simulink library "aerolibwind"  (Simulink 5.0)
libraries: simulink x2, aerolibutil x1
settings Model: ForwardingTableString=||__slOldName__||aerolibwind/Dryden Wind Turbulence Model||__slNewName__||aerolibprivatev1p5/Dryden Wind Turbulence Model||__slOldName__||aerolibwind/Discrete Wind Gust Model||__slNewName__||aerolibprivatev1p5/Discrete Wind Gust Model||__slOldName__||aerolibwind/Wind Shear Model||__slNewName__||aerolibprivatev1p5/Wind Shear Model  Creator=sgage  LastModifiedBy=sgage  ExtModeAutoUpdateStatusClock=off  TargetHWChar=2  TargetHWWordLengths=8,16,32,32

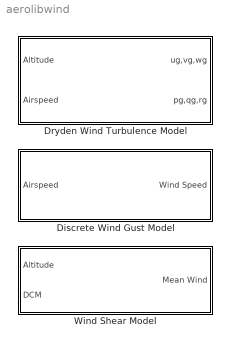
== system aerolibwind ==
  Discrete Wind Gust Model : Subsystem  mask(Discrete Wind Gust Model){v_units=meters/second, Gx=on, Gy=on, Gz=on, t_0=5, d_m=[120 120 80], v_m=[3.5 3.5 3.0]}
      mask prompts: v_units "Units of velocity:"; Gx "Check for gust in u-axis"; Gy "Check for gust in v-axis"; Gz "Check for gust in w-axis"; t_0 "Gust start time (seconds):"; d_m "Gust length [dx dy dz] (meters):"; v_m "Gust amplitude [ug vg wg] (meters/second):"
      mask help: Generate a discrete wind gust. The gust profile takes the '1-cosine' form.
      mask init:
      | m2ft= 3.28084;
      | mps2knot=1.94384;
      | if strcmp(v_units, 'meters/second')
      |   gust_units=1;
      |   mask_text1='m';
      |   mask_text2='m/s';
      | elseif strcmp(v_units, 'feet/second')
      |   gust_units=1;
      |   mask_text1='ft';
      |   mask_text2='ft/s';
      | else
      |   gust_units=m2ft/mps2knot;
      |   mask_text1='ft';
      |   mask_text2='knots';
      | end
      mask Help: web(asbhelp);
      mask StyleString: popup(meters/second|feet/second|knots),checkbox,checkbox,checkbox,edit,edit,edit
      mask CallbackString: aeroicon('aeroblkwindgust')||||||
      mask Display:
      | port_label('output', 1, ['Wind velocity (', mask_text2, ')'])
      | port_label('input', 1, ['Airspeed (', mask_text2, ')'])
  Dryden Wind Turbulence Model : Subsystem  mask(Dryden Wind Turbulence Model){v_units=meters/second, W20=15, TurbProb=10^-2 - Light, L_high=533, Wingspan=10, ts=0.1, Seed=[23341 23342 23343 23344], T_on=on}
      mask prompts: v_units "Units of velocity:"; W20 "Wind speed at 6 m defines the low-altitude intensity (meters/second):"; TurbProb "Probability of exceedance of high-altitude intensity"; L_high "Scale length at medium/high altitudes (meters):"; Wingspan "Wingspan (meters):"; ts "Band-limited noise sample time (seconds):"; Seed "Noise seeds [ug vg wg pg]:"; T_on "Turbulence on"
      mask help: Generate atmospheric turbulence. White noise is passed through a filter to give the turbulence the Dryden velocity spectra.
      mask init:
      | h_vec = [.5 1.75 3.75 7.5 15 25 35 45 55 65 75 80]*1000;% feet
      | sigma_vec(1,:) = [3.2 2.2 1.5 zeros(1,9)]; % ft/sec
      | sigma_vec(2,:) = [4.2 3.6 3.3 1.6 zeros(1,8)];
      | sigma_vec(3,:) = [6.6 6.9 7.4 6.7 4.6 2.7 0.4 zeros(1,5)];
      | sigma_vec(4,:) = [8.6 9.6 10.6 10.1 8.0 6.6 5.0 4.2 2.7 zeros(1,3)];
      | sigma_vec(5,:) = [11.8 13.0 16.0 15.1 11.6 9.7 8.1 8.2 7.9 4.9 3.2 2.1];
      | sigma_vec(6,:) = [15.6 17.6 23.0 23.6 22.1 20.0 16.0 15.1 12.1 7.9 6.2 5.1];
      | sigma_vec(7,:) = [18.7 21.5 28.4 30.2 30.7 31.0 25.2 23.1 17.5 10.7 8.4 7.2];
      | m2ft= 3.28084;
      | mps2knot=1.94384;
      | max_height_low = 1000;
      | min_height_high = 2000;
      | if strcmp(v_units, 'meters/second')
      |     gust_units=1;
      |     alt_units = m2ft;
      |     mask_text1='m';
      |     mask_text2='m/s';
      |     h_vec = h_vec/m2ft;
      |     sigma_vec = sigma_vec/m2ft;
      |     max_height_low = 1000/m2ft;
      |     min_height_high = 2000/m2ft;
      | elseif strcmp(v_units, 'feet/second')
      |     gust_units=1;
      |     alt_units =1;
      |     mask_text1='ft';
      |     mask_text2='ft/s';
      | else
      |     gust_units=m2ft/mps2knot;
      |     alt_units=1;
      |     mask_text1='ft';
      |     mask_text2='knots';
      | end
      mask Help: web(asbhelp);
      mask StyleString: popup(meters/second|feet/second|knots),edit,popup(2x10^-1|10^-1|10^-2 - Light |10^-3 - Moderate|10^-4|10^-5 - Severe|10^-6),edit,edit,edit,edit,checkbox
      mask CallbackString: aeroicon('aeroblkwindturb')|||||||
      mask Display:
      | port_label('output', 1, [' Wind velocity  (', mask_text2, ')'])
      | port_label('output', 2, 'Angular rates (rad/sec)')
      | port_label('input', 1, ['Altitude (', mask_text1, ')'])
      | port_label('input', 2, ['Airspeed (', mask_text2, ')'])
  Wind Shear Model : Subsystem  mask(Wind Shear Model){v_units=meters/second, phase=Category C - Terminal Flight Phase, W_20=15, Wdeg=0}
      mask prompts: v_units "Units of velocity:"; phase "Flight phase:"; W_20 "Wind speed at 6 meters altitude (meters/second):"; Wdeg "Wind direction at 6 meters altitude (degrees clockwise from north):"
      mask help: Calculate the wind shear from conditions measured at a height of 6 meters (20 feet) above the ground.
      mask init:
      | m2ft= 3.28084;
      | if strcmp(v_units, 'meters/second')
      |   if phase == 1;z0 = 0.15/m2ft;else;z0=2.0/m2ft;end;
      |   min_height = 3/m2ft;
      |   ref_height = 6;
      |   mask_text1='m';
      |   mask_text2='m/s';
      | elseif strcmp(v_units, 'feet/second')
      |   if phase == 1;z0 = 0.15;else;z0=2.0;end;
      |   min_height = 3;
      |   ref_height = 20;
      |   mask_text1='ft';
      |   mask_text2='ft/s';
      | else
      |   if phase == 1;z0 = 0.15;else;z0=2.0;end;
      |   min_height = 3;
      |   ref_height = 20;
      |   mask_text1='ft';
      |   mask_text2='knots';
      | end
      mask Help: web(asbhelp);
      mask StyleString: popup(meters/second|feet/second|knots),popup(Category C - Terminal Flight Phase|Other),edit,edit
      mask CallbackString: aeroicon('aeroblkwindshear')|||
      mask Display:
      | port_label('output', 1, ['Wind velocity (', mask_text2, ')'])
      | port_label('input', 1, ['Altitude (', mask_text1, ')'])
      | port_label('input', 2, 'DCM')

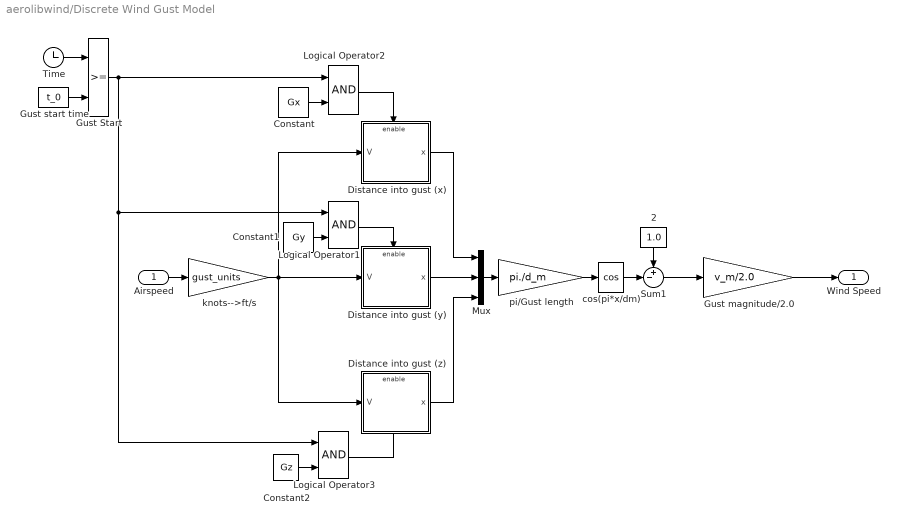
== system aerolibwind/Discrete Wind Gust Model ==
  Airspeed : Inport
  2 : Constant  Orientation=down  Value=1.0
  Constant : Constant  Value=Gx
  Constant1 : Constant  Value=Gy
  Constant2 : Constant  Value=Gz
  Distance into gust (x) : Subsystem  TreatAsAtomicUnit=on  mask{d_m=d_m(1)}
      mask prompts: d_m "Gust length d:"
  Distance into gust (y) : Subsystem  TreatAsAtomicUnit=on  mask{d_m=d_m(2)}
      mask prompts: d_m "Gust length d:"
  Distance into gust (z) : Subsystem  TreatAsAtomicUnit=on  mask{d_m=d_m(3)}
      mask prompts: d_m "Gust length d:"
  Gust Start : RelationalOperator  ShowAdditionalParam=on  LogicOutDataTypeMode=Specify via dialog  LogicDataType=float('double')  InputSameDT=on
  Gust magnitude/2.0 : Gain  Gain=v_m/2.0  SaturateOnIntegerOverflow=on
  Gust start time : Constant  Value=t_0
  Logical Operator1 : Logic  ShowAdditionalParam=on  AllPortsSameDT=off
  Logical Operator2 : Logic  ShowAdditionalParam=on  AllPortsSameDT=off
  Logical Operator3 : Logic  ShowAdditionalParam=on  AllPortsSameDT=off
  Mux : Mux  Inputs=3
  Sum1 : Sum  Inputs=+-|  SaturateOnIntegerOverflow=on  InputSameDT=on
  Time : Clock
      settings: Decimation=10
  cos(pi*x/dm) : Trigonometry  Operator=cos
  knots-->ft/s : Gain  Gain=gust_units  SaturateOnIntegerOverflow=on
  pi/Gust length : Gain  Gain=pi./d_m  SaturateOnIntegerOverflow=on
  Wind Speed : Outport
  wires:
  knots-->ft/s/1 -> Distance into gust (z)/1(V), Distance into gust (x)/1(V), Distance into gust (y)/1(V)
  Distance into gust (x)/1(x) -> Mux/1
  Constant/1 -> Logical Operator2/2
  Gust Start/1 -> Logical Operator2/1, Logical Operator3/1, Logical Operator1/1
  Airspeed/1 -> knots-->ft/s/1
  Logical Operator2/1 -> Distance into gust (x)/Enable
  Constant1/1 -> Logical Operator1/2
  Logical Operator1/1 -> Distance into gust (y)/Enable
  Constant2/1 -> Logical Operator3/2
  Logical Operator3/1 -> Distance into gust (z)/Enable
  Mux/1 -> pi/Gust length/1
  Distance into gust (z)/1(x) -> Mux/3
  Distance into gust (y)/1(x) -> Mux/2
  Gust start time/1 -> Gust Start/2
  Time/1 -> Gust Start/1
  Gust magnitude/2.0/1 -> Wind Speed/1
  cos(pi*x/dm)/1 -> Sum1/2
  Sum1/1 -> Gust magnitude/2.0/1
  2/1 -> Sum1/1
  pi/Gust length/1 -> cos(pi*x/dm)/1

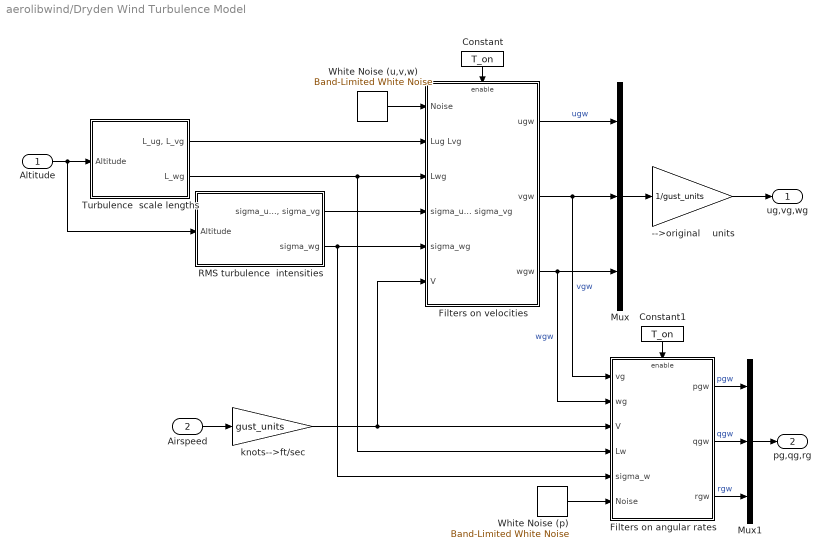
== system aerolibwind/Dryden Wind Turbulence Model ==
  Altitude : Inport
  Airspeed : Inport  Port=2
  -->original    units : Gain  Gain=1/gust_units  SaturateOnIntegerOverflow=on
  Constant : Constant  Orientation=down  Value=T_on
  Constant1 : Constant  Orientation=down  Value=T_on
  Filters on angular rates : Subsystem  TreatAsAtomicUnit=on
  Filters on velocities : Subsystem  TreatAsAtomicUnit=on
  Mux : Mux  Inputs=3
  Mux1 : Mux  Inputs=3
  RMS turbulence  intensities : Subsystem
  Turbulence  scale lengths : Subsystem
  White Noise (p) : simulink/Sources/Band-Limited White Noise  Cov=1  Ts=ts  seed=Seed(4)
  White Noise (u,v,w) : simulink/Sources/Band-Limited White Noise  Cov=[1 1 1]  Ts=ts  seed=Seed(1:3)
  knots-->ft/sec : Gain  Gain=gust_units  SaturateOnIntegerOverflow=on
  ug,vg,wg : Outport
  pg,qg,rg : Outport  Port=2
  wires:
  Constant1/1 -> Filters on angular rates/Enable
  Constant/1 -> Filters on velocities/Enable
  Filters on velocities/3(wgw) -> Filters on angular rates/2(wg), Mux/3  "wgw"
  Filters on velocities/2(vgw) -> Filters on angular rates/1(vg), Mux/2  "vgw"
  RMS turbulence  intensities/1("sigma_ug, sigma_vg ") -> Filters on velocities/4(sigma_ug sigma_vg)
  Filters on velocities/1(ugw) -> Mux/1  "ugw"
  Filters on angular rates/3(rgw) -> Mux1/3  "rgw"
  Filters on angular rates/2(qgw) -> Mux1/2  "qgw"
  Filters on angular rates/1(pgw) -> Mux1/1  "pgw"
  Mux1/1 -> pg,qg,rg/1
  Mux/1 -> -->original    units/1
  RMS turbulence  intensities/2(sigma_wg) -> Filters on velocities/5(sigma_wg), Filters on angular rates/5(sigma_w)
  Turbulence  scale lengths/2(L_wg) -> Filters on angular rates/4(Lw), Filters on velocities/3(Lwg)
  Turbulence  scale lengths/1("L_ug, L_vg") -> Filters on velocities/2(Lug Lvg)
  knots-->ft/sec/1 -> Filters on angular rates/3(V), Filters on velocities/6(V)
  Airspeed/1 -> knots-->ft/sec/1
  Altitude/1 -> RMS turbulence  intensities/1(Altitude), Turbulence  scale lengths/1(Altitude)
  -->original    units/1 -> ug,vg,wg/1
  White Noise (u,v,w)/1 -> Filters on velocities/1(Noise)
  White Noise (p)/1 -> Filters on angular rates/6(Noise)

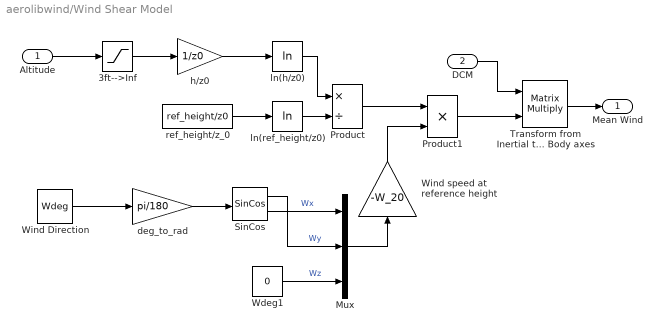
== system aerolibwind/Wind Shear Model ==
  Altitude : Inport
  DCM : Inport  Port=2
  3ft-->Inf : Saturate  UpperLimit=inf  LowerLimit=min_height
  Mux : Mux  Inputs=3
  Product : Product  Inputs=*/  SaturateOnIntegerOverflow=on  InputSameDT=on
  Product1 : Product  SaturateOnIntegerOverflow=on  InputSameDT=on
  SinCos : aerolibutil/SinCos
  Transform from Inertial to Body axes : Product  Inputs=**  Multiplication=Matrix(*)  SaturateOnIntegerOverflow=on  InputSameDT=on
  Wdeg1 : Constant  Value=0
  Wind Direction : Constant  Value=Wdeg
  Wind speed at reference height : Gain  Orientation=up  Gain=-W_20  SaturateOnIntegerOverflow=on
  deg_to_rad : Gain  Gain=pi/180  SaturateOnIntegerOverflow=on
  h/z0 : Gain  Gain=1/z0  SaturateOnIntegerOverflow=on
  ln(h/z0) : Math  Operator=log
  ln(ref_height/z0) : Math  Operator=log
  ref_height/z_0 : Constant  Value=ref_height/z0
  Mean Wind : Outport
  wires:
  Altitude/1 -> 3ft-->Inf/1
  Product/1 -> Product1/1
  ln(ref_height/z0)/1 -> Product/2
  ln(h/z0)/1 -> Product/1
  ref_height/z_0/1 -> ln(ref_height/z0)/1
  h/z0/1 -> ln(h/z0)/1
  3ft-->Inf/1 -> h/z0/1
  Transform from Inertial to Body axes/1 -> Mean Wind/1
  Wind Direction/1 -> deg_to_rad/1
  SinCos/2 -> Mux/1  "Wx"
  SinCos/1 -> Mux/2  "Wy"
  deg_to_rad/1 -> SinCos/1
  Wdeg1/1 -> Mux/3  "Wz"
  Mux/1 -> Wind speed at reference height/1
  Product1/1 -> Transform from Inertial to Body axes/2
  DCM/1 -> Transform from Inertial to Body axes/1
  Wind speed at reference height/1 -> Product1/2

== system aerolibwind/Discrete Wind Gust Model/Distance into gust (x) ==
  V : Inport
  Enable : EnablePort  StatesWhenEnabling=reset
  Distance into Gust (x) (Limited to gust length d) : Integrator  LimitOutput=on  UpperSaturationLimit=d_m  LowerSaturationLimit=0
  x : Outport  InitialOutput=[0]
  wires:
  Distance into Gust (x) (Limited to gust length d)/1 -> x/1
  V/1 -> Distance into Gust (x) (Limited to gust length d)/1

== system aerolibwind/Discrete Wind Gust Model/Distance into gust (y) ==
  V : Inport
  Enable : EnablePort  StatesWhenEnabling=reset
  "Distance into Gust (x) (Limited to gust length d) " : Integrator  LimitOutput=on  UpperSaturationLimit=d_m  LowerSaturationLimit=0
  x : Outport  InitialOutput=[0]
  wires:
  "Distance into Gust (x) (Limited to gust length d) "/1 -> x/1
  V/1 -> "Distance into Gust (x) (Limited to gust length d) "/1

== system aerolibwind/Discrete Wind Gust Model/Distance into gust (z) ==
  V : Inport
  Enable : EnablePort  StatesWhenEnabling=reset
  "Distance into Gust (x) (Limited to gust length d) " : Integrator  LimitOutput=on  UpperSaturationLimit=d_m  LowerSaturationLimit=0
  x : Outport  InitialOutput=[0]
  wires:
  V/1 -> "Distance into Gust (x) (Limited to gust length d) "/1
  "Distance into Gust (x) (Limited to gust length d) "/1 -> x/1

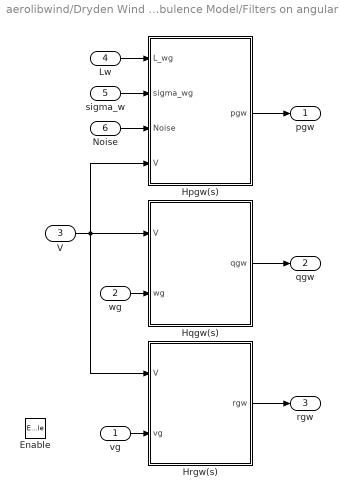
== system aerolibwind/Dryden Wind Turbulence Model/Filters on angular rates ==
  vg : Inport
  wg : Inport  Port=2
  V : Inport  Port=3
  Lw : Inport  Port=4
  sigma_w : Inport  Port=5
  Noise : Inport  Port=6
  Enable : EnablePort  StatesWhenEnabling=reset
  Hpgw(s) : Subsystem
  Hqgw(s) : Subsystem
  Hrgw(s) : Subsystem
  pgw : Outport  OutputWhenDisabled=reset  InitialOutput=0
  qgw : Outport  Port=2  OutputWhenDisabled=reset  InitialOutput=0
  rgw : Outport  Port=3  OutputWhenDisabled=reset  InitialOutput=0
  wires:
  vg/1 -> Hrgw(s)/2(vg)
  Hrgw(s)/1(rgw) -> rgw/1
  Hqgw(s)/1(qgw) -> qgw/1
  wg/1 -> Hqgw(s)/2(wg)
  Hpgw(s)/1(pgw) -> pgw/1
  V/1 -> Hqgw(s)/1(V), Hrgw(s)/1(V), Hpgw(s)/4(V)
  sigma_w/1 -> Hpgw(s)/2(sigma_wg)
  Lw/1 -> Hpgw(s)/1(L_wg)
  Noise/1 -> Hpgw(s)/3(Noise)

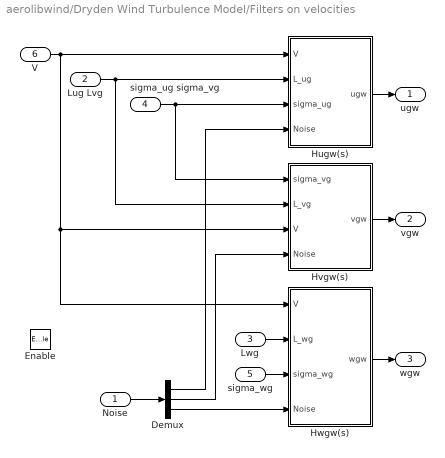
== system aerolibwind/Dryden Wind Turbulence Model/Filters on velocities ==
  Noise : Inport
  Lug Lvg : Inport  Port=2
  Lwg : Inport  Port=3
  sigma_ug sigma_vg : Inport  Port=4
  sigma_wg : Inport  Port=5
  V : Inport  Port=6
  Enable : EnablePort  StatesWhenEnabling=reset
  Demux : Demux  Outputs=3
  Hugw(s) : Subsystem
  Hvgw(s) : Subsystem
  Hwgw(s) : Subsystem
  ugw : Outport  OutputWhenDisabled=reset  InitialOutput=0
  vgw : Outport  Port=2  OutputWhenDisabled=reset  InitialOutput=0
  wgw : Outport  Port=3  OutputWhenDisabled=reset  InitialOutput=0
  wires:
  sigma_wg/1 -> Hwgw(s)/3(sigma_wg)
  Lwg/1 -> Hwgw(s)/2(L_wg)
  sigma_ug sigma_vg/1 -> Hvgw(s)/1(sigma_vg), Hugw(s)/3(sigma_ug)
  Lug Lvg/1 -> Hvgw(s)/2(L_vg), Hugw(s)/2(L_ug)
  V/1 -> Hwgw(s)/1(V), Hvgw(s)/3(V), Hugw(s)/1(V)
  Demux/3 -> Hwgw(s)/4(Noise)
  Hugw(s)/1(ugw) -> ugw/1
  Hvgw(s)/1(vgw) -> vgw/1
  Hwgw(s)/1(wgw) -> wgw/1
  Noise/1 -> Demux/1
  Demux/1 -> Hugw(s)/4(Noise)
  Demux/2 -> Hvgw(s)/4(Noise)

== system aerolibwind/Dryden Wind Turbulence Model/RMS turbulence  intensities ==
  Altitude : Inport
  High Altitude Intensity : Subsystem  TreatAsAtomicUnit=on
  Interpolate : Subsystem  TreatAsAtomicUnit=on
  Low Altitude Intensity : Subsystem  TreatAsAtomicUnit=on
  Sum : Sum  Inputs=+++  SaturateOnIntegerOverflow=on  InputSameDT=on
  Sum1 : Sum  Inputs=+++  SaturateOnIntegerOverflow=on  InputSameDT=on
  if Height < Max low altitude  elseif Height > Min isotropic altitude : If  IfExpression=u1<=max_height_low  ElseIfExpressions=u1>=min_height_high
  "sigma_ug, sigma_vg " : Outport
  sigma_wg : Outport  Port=2
  wires:
  Sum1/1 -> sigma_wg/1  "sigmawg"
  Interpolate/1(sigma_wg) -> Sum1/3
  Low Altitude Intensity/2(sigma_wg) -> Sum1/1
  Sum/1 -> "sigma_ug, sigma_vg "/1  "sigmaug"
  Interpolate/2(sigma_ug sigma_vg) -> Sum/3
  High Altitude Intensity/1(sigma_ug sigma_vg sigma_wg) -> Sum1/2, Sum/2
  Low Altitude Intensity/1(sigma_ug sigma_vg) -> Sum/1
  Altitude/1 -> Interpolate/1(h), High Altitude Intensity/1(h), if Height < Max low altitude  elseif Height > Min isotropic altitude/1, Low Altitude Intensity/1(h)
  if Height < Max low altitude  elseif Height > Min isotropic altitude/3 -> Interpolate/Action
  if Height < Max low altitude  elseif Height > Min isotropic altitude/2 -> High Altitude Intensity/Action
  if Height < Max low altitude  elseif Height > Min isotropic altitude/1 -> Low Altitude Intensity/Action

== system aerolibwind/Dryden Wind Turbulence Model/Turbulence  scale lengths ==
  Altitude : Inport
  Interpolate : Subsystem  TreatAsAtomicUnit=on
  Low altitude scale length : Subsystem  TreatAsAtomicUnit=on
  Medium/High altitude scale length : Subsystem  TreatAsAtomicUnit=on
  Sum : Sum  Inputs=+++  SaturateOnIntegerOverflow=on  InputSameDT=on
  Sum1 : Sum  Inputs=+++  SaturateOnIntegerOverflow=on  InputSameDT=on
  "if Height < Max low altitude  elseif Height > Min isotropic altitude " : If  IfExpression=u1<=max_height_low  ElseIfExpressions=u1>=min_height_high
  "L_ug, L_vg" : Outport
  L_wg : Outport  Port=2
  wires:
  Altitude/1 -> Low altitude scale length/1(h), Interpolate/1(h), "if Height < Max low altitude  elseif Height > Min isotropic altitude "/1
  "if Height < Max low altitude  elseif Height > Min isotropic altitude "/1 -> Low altitude scale length/Action
  "if Height < Max low altitude  elseif Height > Min isotropic altitude "/2 -> Medium/High altitude scale length/Action
  "if Height < Max low altitude  elseif Height > Min isotropic altitude "/3 -> Interpolate/Action
  Interpolate/2(L_ug L_vg) -> Sum/3
  Interpolate/1(L_wg) -> Sum1/3
  Sum/1 -> L_wg/1  "Lwg"
  Sum1/1 -> "L_ug, L_vg"/1  "Lug"
  Low altitude scale length/1(L_ug L_vg) -> Sum1/1
  Low altitude scale length/2(L_wg) -> Sum/1
  Medium/High altitude scale length/1(L_ug L_vg L_wg) -> Sum/2, Sum1/2

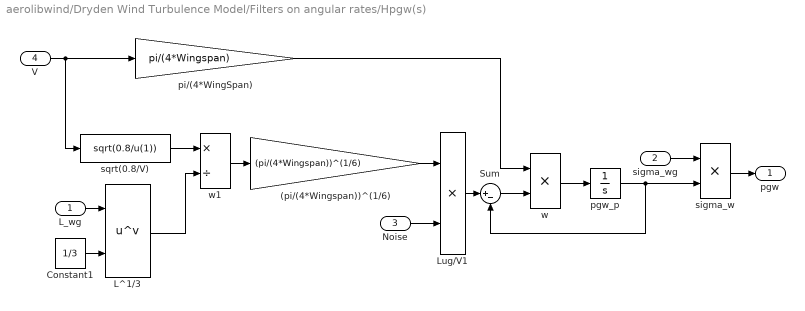
== system aerolibwind/Dryden Wind Turbulence Model/Filters on angular rates/Hpgw(s) ==
  L_wg : Inport
  sigma_wg : Inport  Port=2
  Noise : Inport  Port=3
  V : Inport  Port=4
  (pi/(4*Wingspan))^(1/6) : Gain  Gain=(pi/(4*Wingspan))^(1/6)  SaturateOnIntegerOverflow=on
  Constant1 : Constant  Value=1/3
  L^1/3 : Math  Operator=pow
  Lug/V1 : Product  SaturateOnIntegerOverflow=on  InputSameDT=on
  Sum : Sum  Inputs=|+-  SaturateOnIntegerOverflow=on  InputSameDT=on
  pgw_p : Integrator
  pi/(4*WingSpan) : Gain  Gain=pi/(4*Wingspan)  SaturateOnIntegerOverflow=on
  sigma_w : Product  SaturateOnIntegerOverflow=on  InputSameDT=on
  sqrt(0.8/V) : Fcn  Expr=sqrt(0.8/u(1))
  w : Product  SaturateOnIntegerOverflow=on  InputSameDT=on
  w1 : Product  Inputs=*/  SaturateOnIntegerOverflow=on  InputSameDT=on
  pgw : Outport  InitialOutput=0
  wires:
  w1/1 -> (pi/(4*Wingspan))^(1/6)/1
  (pi/(4*Wingspan))^(1/6)/1 -> Lug/V1/1
  L^1/3/1 -> w1/2
  Noise/1 -> Lug/V1/2
  sqrt(0.8/V)/1 -> w1/1
  L_wg/1 -> L^1/3/1
  sigma_wg/1 -> sigma_w/1
  sigma_w/1 -> pgw/1
  pi/(4*WingSpan)/1 -> w/1
  Constant1/1 -> L^1/3/2
  pgw_p/1 -> sigma_w/2, Sum/2
  V/1 -> sqrt(0.8/V)/1, pi/(4*WingSpan)/1
  w/1 -> pgw_p/1
  Lug/V1/1 -> Sum/1
  Sum/1 -> w/2

== system aerolibwind/Dryden Wind Turbulence Model/Filters on angular rates/Hqgw(s) ==
  V : Inport
  wg : Inport  Port=2
  Sum : Sum  Inputs=|+-  SaturateOnIntegerOverflow=on  InputSameDT=on
  pi/(4*WingSpan) : Gain  Gain=pi/(4*Wingspan)  SaturateOnIntegerOverflow=on
  qgw_p : Integrator
  w : Product  SaturateOnIntegerOverflow=on  InputSameDT=on
  wg/V : Product  Inputs=/*  SaturateOnIntegerOverflow=on  InputSameDT=on
  qgw : Outport  InitialOutput=0
  wires:
  wg/1 -> wg/V/2
  wg/V/1 -> Sum/1
  Sum/1 -> w/2
  w/1 -> qgw/1, qgw_p/1
  V/1 -> wg/V/1, pi/(4*WingSpan)/1
  qgw_p/1 -> Sum/2
  pi/(4*WingSpan)/1 -> w/1

== system aerolibwind/Dryden Wind Turbulence Model/Filters on angular rates/Hrgw(s) ==
  V : Inport
  vg : Inport  Port=2
  -1 : Gain  Gain=-1  SaturateOnIntegerOverflow=on
  Sum : Sum  Inputs=|+-  SaturateOnIntegerOverflow=on  InputSameDT=on
  pi/(4*WingSpan) : Gain  Gain=pi/(3*Wingspan)  SaturateOnIntegerOverflow=on
  rgw_p : Integrator
  vg/V : Product  Inputs=/*  SaturateOnIntegerOverflow=on  InputSameDT=on
  w : Product  SaturateOnIntegerOverflow=on  InputSameDT=on
  rgw : Outport  InitialOutput=0
  wires:
  -1/1 -> rgw/1
  vg/V/1 -> Sum/1
  vg/1 -> vg/V/2
  pi/(4*WingSpan)/1 -> w/1
  rgw_p/1 -> Sum/2
  V/1 -> vg/V/1, pi/(4*WingSpan)/1
  w/1 -> -1/1, rgw_p/1
  Sum/1 -> w/2

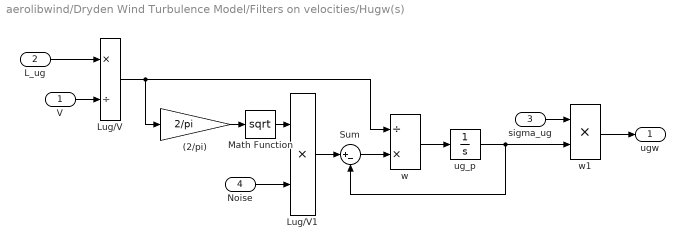
== system aerolibwind/Dryden Wind Turbulence Model/Filters on velocities/Hugw(s) ==
  V : Inport
  L_ug : Inport  Port=2
  sigma_ug : Inport  Port=3
  Noise : Inport  Port=4
  (2/pi) : Gain  Gain=2/pi  SaturateOnIntegerOverflow=on
  Lug/V : Product  Inputs=*/  SaturateOnIntegerOverflow=on  InputSameDT=on
  Lug/V1 : Product  SaturateOnIntegerOverflow=on  InputSameDT=on
  Math Function : Math  Operator=sqrt
  Sum : Sum  Inputs=|+-  SaturateOnIntegerOverflow=on  InputSameDT=on
  ug_p : Integrator
  w : Product  Inputs=/*  SaturateOnIntegerOverflow=on  InputSameDT=on
  w1 : Product  SaturateOnIntegerOverflow=on  InputSameDT=on
  ugw : Outport  InitialOutput=0
  wires:
  Math Function/1 -> Lug/V1/1
  (2/pi)/1 -> Math Function/1
  Noise/1 -> Lug/V1/2
  sigma_ug/1 -> w1/1
  w1/1 -> ugw/1
  ug_p/1 -> w1/2, Sum/2
  L_ug/1 -> Lug/V/1
  V/1 -> Lug/V/2
  w/1 -> ug_p/1
  Lug/V1/1 -> Sum/1
  Sum/1 -> w/2
  Lug/V/1 -> (2/pi)/1, w/1

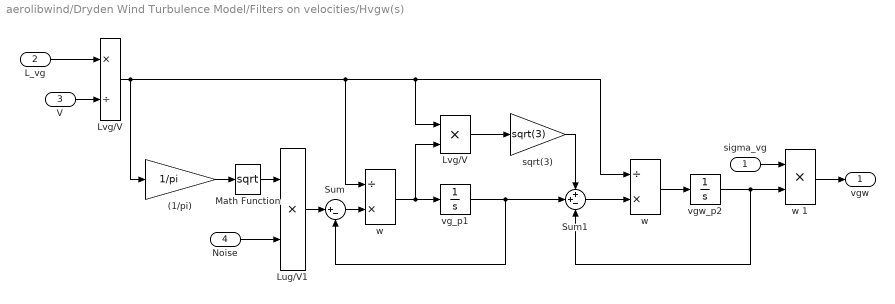
== system aerolibwind/Dryden Wind Turbulence Model/Filters on velocities/Hvgw(s) ==
  sigma_vg : Inport
  L_vg : Inport  Port=2
  V : Inport  Port=3
  Noise : Inport  Port=4
  (1/pi) : Gain  Gain=1/pi  SaturateOnIntegerOverflow=on
  Lug/V1 : Product  SaturateOnIntegerOverflow=on  InputSameDT=on
  Lvg/V : Product  Inputs=*/  SaturateOnIntegerOverflow=on  InputSameDT=on
  "Lvg/V " : Product  SaturateOnIntegerOverflow=on  InputSameDT=on
  Math Function : Math  Operator=sqrt
  Sum : Sum  Inputs=|+-  SaturateOnIntegerOverflow=on  InputSameDT=on
  Sum1 : Sum  Inputs=++-  SaturateOnIntegerOverflow=on  InputSameDT=on
  sqrt(3) : Gain  Gain=sqrt(3)  SaturateOnIntegerOverflow=on
  vg_p1 : Integrator
  vgw_p2 : Integrator
  w : Product  Inputs=/*  SaturateOnIntegerOverflow=on  InputSameDT=on
  "w " : Product  Inputs=/*  SaturateOnIntegerOverflow=on  InputSameDT=on
  w 1 : Product  SaturateOnIntegerOverflow=on  InputSameDT=on
  vgw : Outport  InitialOutput=0
  wires:
  Math Function/1 -> Lug/V1/1
  w 1/1 -> vgw/1
  Noise/1 -> Lug/V1/2
  sigma_vg/1 -> w 1/1
  Lvg/V/1 -> (1/pi)/1, w/1, "w "/1, "Lvg/V "/1
  Sum/1 -> w/2
  Lug/V1/1 -> Sum/1
  w/1 -> vg_p1/1, "Lvg/V "/2
  V/1 -> Lvg/V/2
  L_vg/1 -> Lvg/V/1
  vg_p1/1 -> Sum/2, Sum1/2
  vgw_p2/1 -> w 1/2, Sum1/3
  Sum1/1 -> "w "/2
  "w "/1 -> vgw_p2/1
  "Lvg/V "/1 -> sqrt(3)/1
  sqrt(3)/1 -> Sum1/1
  (1/pi)/1 -> Math Function/1

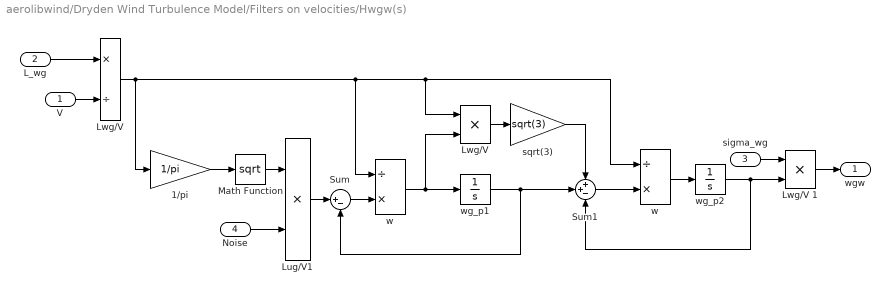
== system aerolibwind/Dryden Wind Turbulence Model/Filters on velocities/Hwgw(s) ==
  V : Inport
  L_wg : Inport  Port=2
  sigma_wg : Inport  Port=3
  Noise : Inport  Port=4
  1/pi : Gain  Gain=1/pi  SaturateOnIntegerOverflow=on
  Lug/V1 : Product  SaturateOnIntegerOverflow=on  InputSameDT=on
  Lwg/V : Product  Inputs=*/  SaturateOnIntegerOverflow=on  InputSameDT=on
  "Lwg/V " : Product  SaturateOnIntegerOverflow=on  InputSameDT=on
  Lwg/V 1 : Product  SaturateOnIntegerOverflow=on  InputSameDT=on
  Math Function : Math  Operator=sqrt
  Sum : Sum  Inputs=|+-  SaturateOnIntegerOverflow=on  InputSameDT=on
  Sum1 : Sum  Inputs=++-  SaturateOnIntegerOverflow=on  InputSameDT=on
  sqrt(3) : Gain  Gain=sqrt(3)  SaturateOnIntegerOverflow=on
  w : Product  Inputs=/*  SaturateOnIntegerOverflow=on  InputSameDT=on
  "w " : Product  Inputs=/*  SaturateOnIntegerOverflow=on  InputSameDT=on
  wg_p1 : Integrator
  wg_p2 : Integrator
  wgw : Outport  InitialOutput=0
  wires:
  1/pi/1 -> Math Function/1
  Noise/1 -> Lug/V1/2
  sigma_wg/1 -> Lwg/V 1/1
  Lwg/V 1/1 -> wgw/1
  "Lwg/V "/1 -> sqrt(3)/1
  "w "/1 -> wg_p2/1
  Sum1/1 -> "w "/2
  wg_p2/1 -> Lwg/V 1/2, Sum1/3
  wg_p1/1 -> Sum1/2, Sum/2
  L_wg/1 -> Lwg/V/1
  V/1 -> Lwg/V/2
  w/1 -> wg_p1/1, "Lwg/V "/2
  Lug/V1/1 -> Sum/1
  Sum/1 -> w/2
  Lwg/V/1 -> 1/pi/1, "Lwg/V "/1, "w "/1, w/1
  Math Function/1 -> Lug/V1/1
  sqrt(3)/1 -> Sum1/1

== system aerolibwind/Dryden Wind Turbulence Model/RMS turbulence  intensities/High Altitude Intensity ==
  h : Inport
  Action Port : ActionPort
  Gain : Gain  SaturateOnIntegerOverflow=on
  Limit height to table : Saturate  UpperLimit=max(h_vec)  LowerLimit=min(h_vec)
  Medium/High Altitude Intensity : Lookup2D  RowIndex=h_vec  ColumnIndex=[1:7]  OutputValues=sigma_vec'  SaturateOnIntegerOverflow=on  InputSameDT=on
  Probability of  Exceedance : Constant  Value=TurbProb
  sigma_ug sigma_vg sigma_wg : Outport  OutputWhenDisabled=reset  InitialOutput=0
  wires:
  h/1 -> Limit height to table/1
  Medium/High Altitude Intensity/1 -> sigma_ug sigma_vg sigma_wg/1
  Probability of  Exceedance/1 -> Medium/High Altitude Intensity/2
  Limit height to table/1 -> Gain/1
  Gain/1 -> Medium/High Altitude Intensity/1

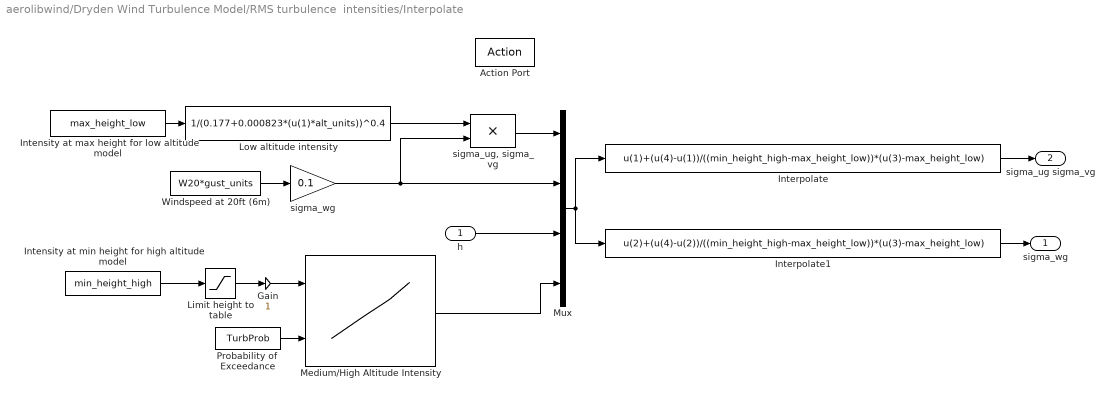
== system aerolibwind/Dryden Wind Turbulence Model/RMS turbulence  intensities/Interpolate ==
  h : Inport
  Action Port : ActionPort
  Gain : Gain  SaturateOnIntegerOverflow=on
  Intensity at max height for low altitude model : Constant  Value=max_height_low
  Intensity at min height for high altitude model : Constant  Value=min_height_high
  Interpolate : Fcn  Expr=u(1)+(u(4)-u(1))/((min_height_high-max_height_low))*(u(3)-max_height_low)
  Interpolate1 : Fcn  Expr=u(2)+(u(4)-u(2))/((min_height_high-max_height_low))*(u(3)-max_height_low)
  Limit height to table : Saturate  UpperLimit=max(h_vec)  LowerLimit=min(h_vec)
  Low altitude intensity : Fcn  Expr=1/(0.177+0.000823*(u(1)*alt_units))^0.4
  Medium/High Altitude Intensity : Lookup2D  RowIndex=h_vec  ColumnIndex=[1:7]  OutputValues=sigma_vec'  SaturateOnIntegerOverflow=on  InputSameDT=on
  Mux : Mux
  Probability of  Exceedance : Constant  Value=TurbProb
  Windspeed at 20ft (6m) : Constant  Value=W20*gust_units
  "sigma_ug, sigma_vg" : Product  SaturateOnIntegerOverflow=on  InputSameDT=on
  "sigma_wg " : Gain  Gain=0.1  SaturateOnIntegerOverflow=on
  sigma_wg : Outport  OutputWhenDisabled=reset  InitialOutput=0
  sigma_ug sigma_vg : Outport  Port=2  OutputWhenDisabled=reset  InitialOutput=0
  wires:
  Interpolate1/1 -> sigma_wg/1
  Interpolate/1 -> sigma_ug sigma_vg/1
  Mux/1 -> Interpolate1/1, Interpolate/1
  h/1 -> Mux/3
  "sigma_ug, sigma_vg"/1 -> Mux/1
  Intensity at max height for low altitude model/1 -> Low altitude intensity/1
  Low altitude intensity/1 -> "sigma_ug, sigma_vg"/1
  "sigma_wg "/1 -> Mux/2, "sigma_ug, sigma_vg"/2
  Windspeed at 20ft (6m)/1 -> "sigma_wg "/1
  Probability of  Exceedance/1 -> Medium/High Altitude Intensity/2
  Intensity at min height for high altitude model/1 -> Limit height to table/1
  Medium/High Altitude Intensity/1 -> Mux/4
  Limit height to table/1 -> Gain/1
  Gain/1 -> Medium/High Altitude Intensity/1

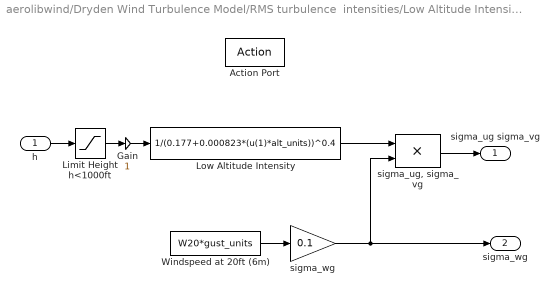
== system aerolibwind/Dryden Wind Turbulence Model/RMS turbulence  intensities/Low Altitude Intensity ==
  h : Inport
  Action Port : ActionPort
  Gain : Gain  SaturateOnIntegerOverflow=on
  Limit Height h<1000ft : Saturate  UpperLimit=max_height_low  LowerLimit=0
  Low Altitude Intensity : Fcn  Expr=1/(0.177+0.000823*(u(1)*alt_units))^0.4
  Windspeed at 20ft (6m) : Constant  Value=W20*gust_units
  "sigma_ug, sigma_vg" : Product  SaturateOnIntegerOverflow=on  InputSameDT=on
  "sigma_wg " : Gain  Gain=0.1  SaturateOnIntegerOverflow=on
  sigma_ug sigma_vg : Outport  OutputWhenDisabled=reset  InitialOutput=0
  sigma_wg : Outport  Port=2  OutputWhenDisabled=reset  InitialOutput=0
  wires:
  "sigma_ug, sigma_vg"/1 -> sigma_ug sigma_vg/1
  h/1 -> Limit Height h<1000ft/1
  Low Altitude Intensity/1 -> "sigma_ug, sigma_vg"/1
  "sigma_wg "/1 -> sigma_wg/1, "sigma_ug, sigma_vg"/2
  Windspeed at 20ft (6m)/1 -> "sigma_wg "/1
  Gain/1 -> Low Altitude Intensity/1
  Limit Height h<1000ft/1 -> Gain/1

== system aerolibwind/Dryden Wind Turbulence Model/Turbulence  scale lengths/Interpolate ==
  h : Inport
  Action Port : ActionPort
  Interpolate : Fcn  Expr=u(1)+(u(4)-u(1))/((min_height_high-max_height_low))*(u(3)-max_height_low)
  Interpolate1 : Fcn  Expr=u(2)+(u(4)-u(2))/((min_height_high-max_height_low))*(u(3)-max_height_low)
  Low Altitude Scale Length : Fcn  Expr=u(1)/(0.177+0.000823*(u(1)*alt_units))^1.2
  Maximum height for low altitude model : Constant  Value=max_height_low
  Medium/High Altitude Scale Length : Constant  Value=L_high
  Mux : Mux
  L_wg : Outport  OutputWhenDisabled=reset  InitialOutput=0
  L_ug L_vg : Outport  Port=2  OutputWhenDisabled=reset  InitialOutput=0
  wires:
  Medium/High Altitude Scale Length/1 -> Mux/4
  Interpolate1/1 -> L_wg/1
  Interpolate/1 -> L_ug L_vg/1
  Mux/1 -> Interpolate1/1, Interpolate/1
  h/1 -> Mux/3
  Maximum height for low altitude model/1 -> Mux/2, Low Altitude Scale Length/1
  Low Altitude Scale Length/1 -> Mux/1

== system aerolibwind/Dryden Wind Turbulence Model/Turbulence  scale lengths/Low altitude scale length ==
  h : Inport
  Action Port : ActionPort
  Gain : Gain  SaturateOnIntegerOverflow=on
  Limit Function 10ft to 1000ft : Saturate  UpperLimit=max_height_low  LowerLimit=10/alt_units
  Low Altitude Scale Length : Fcn  Expr=u(1)/(0.177+0.000823*(u(1)*alt_units))^1.2
  L_ug L_vg : Outport  OutputWhenDisabled=reset  InitialOutput=0
  L_wg : Outport  Port=2  OutputWhenDisabled=reset  InitialOutput=0
  wires:
  h/1 -> Limit Function 10ft to 1000ft/1
  Low Altitude Scale Length/1 -> L_ug L_vg/1
  Limit Function 10ft to 1000ft/1 -> Gain/1
  Gain/1 -> L_wg/1, Low Altitude Scale Length/1

== system aerolibwind/Dryden Wind Turbulence Model/Turbulence  scale lengths/Medium/High altitude scale length ==
  Action Port : ActionPort
  Medium/High Altitude : Constant  Value=L_high
  L_ug L_vg L_wg : Outport  OutputWhenDisabled=reset  InitialOutput=0
  wires:
  Medium/High Altitude/1 -> L_ug L_vg L_wg/1
